simulink model "polar2dec"  (R2020b)
settings: Solver=VariableStepAuto  StartTime=0.0  StopTime=50  RelTol=1e-3
settings Model: Creator=Bk_space  LastModifiedBy=Bk_space

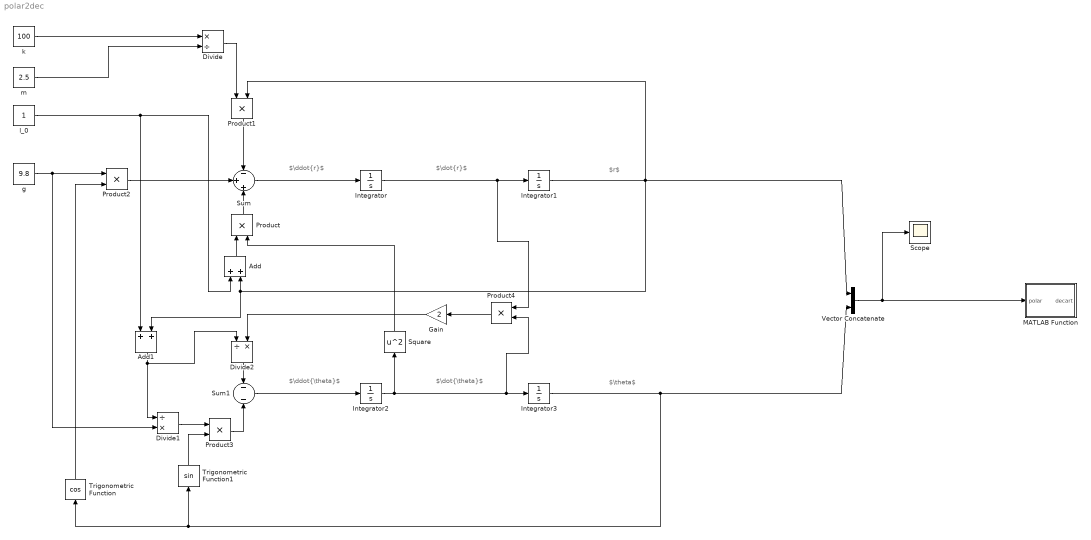
== system polar2dec ==
  note: $r$
  note: $\ddot{r}$
  note: $\dot{r}$
  note: $\theta$
  note: $\ddot{\theta}$
  note: $\dot{\theta}$
  Add : Sum
  Add1 : Sum
  Divide : Product  Inputs=*/
  Divide1 : Product  Inputs=/*
  Divide2 : Product  Inputs=/*
  Gain : Gain  Gain=2
  Integrator : Integrator  InitialCondition=1
  Integrator1 : Integrator  InitialCondition=1
  Integrator2 : Integrator
  Integrator3 : Integrator  InitialCondition=45
  MATLAB Function : MATLAB Function  TreatAsAtomicUnit=on
  Product{,1..4} (5 alike) : Product
  Scope : Scope
  Square : Math  Operator=square  OutputSignalType=real  SaturateOnIntegerOverflow=on
  Sum : Sum  Inputs=-|+|+
  Sum1 : Sum  Inputs=--
  Trigonometric Function : Trigonometry  Operator=cos  OutputSignalType=real
  Trigonometric Function1 : Trigonometry  OutputSignalType=real
  Vector Concatenate : Concatenate
  g : Constant  Value=9.8
  k : Constant  Value=100
  l_0 : Constant
  m : Constant  Value=2.5
  wires:
  Integrator/1 -> Product4/1, Integrator1/1
  Integrator1/1 -> Add1/2, Add/2, Vector Concatenate/1, Product1/2
  Sum/1 -> Integrator/1
  Integrator2/1 -> Product4/2, Integrator3/1, Square/1
  Sum1/1 -> Integrator2/1
  Integrator3/1 -> Vector Concatenate/2, Trigonometric Function/1, Trigonometric Function1/1
  Square/1 -> Product/2
  l_0/1 -> Add/1, Add1/1
  Add/1 -> Product/1
  Product/1 -> Sum/3
  k/1 -> Divide/1
  m/1 -> Divide/2
  Divide/1 -> Product1/1
  Product1/1 -> Sum/1
  Trigonometric Function/1 -> Product2/2
  g/1 -> Product2/1, Divide1/2
  Product2/1 -> Sum/2
  Trigonometric Function1/1 -> Product3/2
  Product3/1 -> Sum1/2
  Add1/1 -> Divide2/1, Divide1/1
  Divide1/1 -> Product3/1
  Divide2/1 -> Sum1/1
  Product4/1 -> Gain/1
  Gain/1 -> Divide2/2
  Vector Concatenate/1 -> MATLAB Function/1(polar), Scope/1

== matlab function polar2dec/MATLAB Function ==
  data: polar input; decart output
function decart = pol2dec(polar)
decart = [1, 2];
decart(1) = polar(1) * sin(polar(2));
decart(2) = - polar(1) * cos(polar(2));
end
